simulink model "main_tmp"  (R2021b)
settings: Solver=VariableStepAuto  StartTime=0.0  StopTime=5  FixedStep=Ts  RelTol=1e-3  AbsTol=1e-3  EnableMultiTasking=on
values from neighbouring files (symbols this model uses):
  N = length(dataset.(fldnames{1}))    [create_timeseries.m]    (also in input_data.m = length(t); test_input_data.m = length(t))
undefined symbols (not defined in the file or in its folder): bodyparam, stuffparam, X, Y, Z
libraries: sm_lib x37, nesl_utility x13, Muscles4SimScienceAB x5, Contact_Forces_Lib x2, simulink x1
(part 2 of 2)

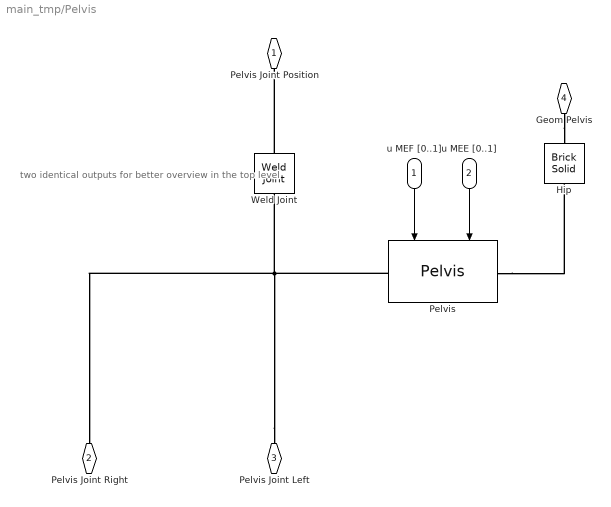
== system main_tmp/Pelvis ==
  note: two identical outputs for better overview in the top level
  u MEF [0..1] : Inport
  u MEE [0..1] : Inport  Port=2
  Hip : sm_lib/Body Elements/Brick Solid  GraphicAmbientColor=[0.15 0.15 0.15 1.0]  BasedOnType=Mass  BrickDimensions=bodyparam.size.hip  BrickDimensionUnits=m  CenterOfMass=[0 0 0]  CenterOfMassUnits=m  GraphicDiffuseColor=[0.5 0.5 0.5]  Density=1000  DensityUnits=kg/m^3  DoExposeReferenceFrame=on  GraphicEmissiveColor=[0.0 0.0 0.0 1.0]  ExportEntireGeometry=on  SerializedFrames=<Frames/>  MarkerShape=Sphere  MarkerSize=10  GraphicType=FromGeometry  InertiaType=Custom  Mass=bodyparam.weight.hip  MassUnits=kg  MomentsOfInertia=[1 1 1]  MomentsOfInertiaUnits=kg*m^2  GraphicOpacity=1.0  ProductsOfInertia=[0 0 0]  ProductsOfInertiaUnits=kg*m^2  GraphicShininess=75  GraphicSpecularColor=[0.5 0.5 0.5 1.0]  GraphicVisPropType=SimpleVisualProperties
  Pelvis : Muscles4SimScienceAB/Pelvis  SystemSampleTime=-1  VariantActivationTime=update diagram  Latency=0  AutoFrameSizeCalculation=off
      settings: SourceProductName=Muscles4SimScienceAB  PortSchema="{\"entries\":[{\"content\":{\"sides\":[{\"content\":{\"connectorIds\":[\"In1\",\"In2\"]},\"type\":\"ConnectorPlacement.EquallySpacedRectSide\",\"uuid\":\"96b1b743-5705-4ec0-abfd-bdeea3d69127\"},{\"content\":{\"connectorIds\":[],\"side\":\"RIGHT\"},\"type\":\"ConnectorPlacement.EquallySpacedRectSide\",\"uuid\":\"b3b1b644-d2fe-42fd-b3a0-cbeacae3e2ea\"},{\"content\":{\"connectorIds\":[\"LConn1\"],\"side\":\"TOP\"},\"type\":\"ConnectorPlacement.EquallySpacedRectSide\",\"uuid\":\"6588cc9c-075c-4f00-8cf7-0671acb35c7c\"},{\"content\":{\"connectorIds\":[\"RConn1\"],\"side\":\"BOTTOM\"},\"type\":\"ConnectorPlacement.EquallySpacedRectSide\",\"uuid\":\"6976fdf2-9376-49cf-8dcb-736f43a1e3aa\"}]},\"type\":\"ConnectorPlacement.EquallySpacedConnector\",\"uuid\":\"9665cf7e-0d90-4f65-9e3e-57dbf89b4304\"}],\"packageUris\":[\"http://schema.mathworks.com/mf0/Connector/R2020b\"],\"version\":\"1.0\"}"
  Weld Joint : sm_lib/Joints/Weld Joint  JointMode=Normal  SenseConstraintForce=off  SenseConstraintForceX=off  SenseConstraintForceY=off  SenseConstraintForceZ=off  SenseConstraintTorque=off  SenseConstraintTorqueX=off  SenseConstraintTorqueY=off  SenseConstraintTorqueZ=off  SenseTotalForce=off  SenseTotalForceX=off  SenseTotalForceY=off  SenseTotalForceZ=off  SenseTotalTorque=off  SenseTotalTorqueX=off  SenseTotalTorqueY=off  SenseTotalTorqueZ=off  CompositeWrenchDir=FollowerOnBase  CompositeWrenchFrame=BaseFrame
  Pelvis Joint Position : PMIOPort  Side=Left
  Pelvis Joint Right : PMIOPort  Port=2  Side=Right
  Pelvis Joint Left : PMIOPort  Port=3  Side=Right
  Geom Pelvis : PMIOPort  Port=4  Side=Right
  wires:
  u MEE [0..1]/1 -> Pelvis/1
  u MEF [0..1]/1 -> Pelvis/2
  connections:
  Weld Joint/RConn1 -- Pelvis Joint Position/RConn1
  Geom Pelvis/RConn1 -- Hip/LConn1
  Pelvis Joint Left/RConn1 -- Pelvis/RConn1 -- Weld Joint/LConn1 -- Pelvis Joint Right/RConn1
  Pelvis/LConn1 -- Hip/RConn1

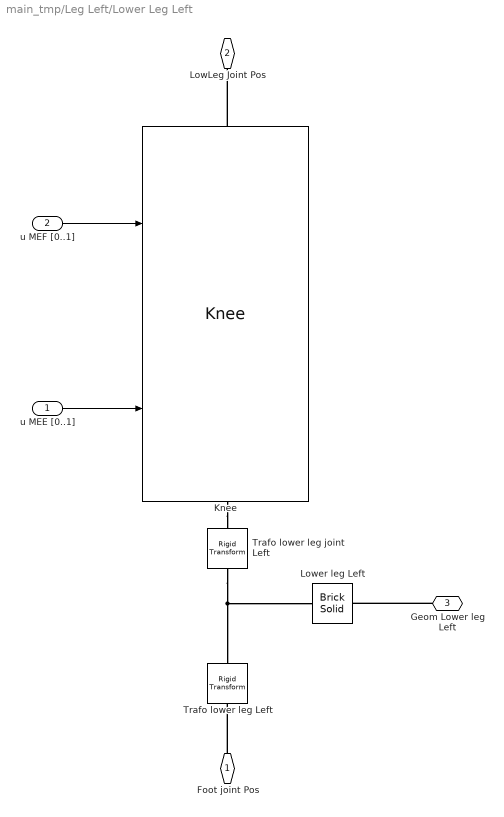
== system main_tmp/Leg Left/Lower Leg Left ==
  u MEE [0..1] : Inport
  u MEF [0..1] : Inport  Port=2
  Knee : Muscles4SimScienceAB/Knee  SystemSampleTime=-1  VariantActivationTime=update diagram  Latency=0  AutoFrameSizeCalculation=off
      settings: SourceProductName=Muscles4SimScienceAB  PortSchema="{\"entries\":[{\"content\":{\"sides\":[{\"content\":{\"connectorIds\":[\"In1\",\"In2\"]},\"type\":\"ConnectorPlacement.EquallySpacedRectSide\",\"uuid\":\"41193043-8a27-4363-8898-1f9e881d08b1\"},{\"content\":{\"connectorIds\":[],\"side\":\"RIGHT\"},\"type\":\"ConnectorPlacement.EquallySpacedRectSide\",\"uuid\":\"5a179196-4a66-423b-80c7-02c9aceed262\"},{\"content\":{\"connectorIds\":[\"LConn1\"],\"side\":\"TOP\"},\"type\":\"ConnectorPlacement.EquallySpacedRectSide\",\"uuid\":\"db447b50-73cc-4af2-8c9c-28a9801561ff\"},{\"content\":{\"connectorIds\":[\"RConn1\"],\"side\":\"BOTTOM\"},\"type\":\"ConnectorPlacement.EquallySpacedRectSide\",\"uuid\":\"bc7ed954-e11d-4420-941c-b14a31097b3c\"}]},\"type\":\"ConnectorPlacement.EquallySpacedConnector\",\"uuid\":\"a73193d2-090f-471b-ad63-2ab894437460\"}],\"packageUris\":[\"http://schema.mathworks.com/mf0/Connector/R2020b\"],\"version\":\"1.0\"}"
  Lower leg Left : sm_lib/Body Elements/Brick Solid  GraphicAmbientColor=[0.15 0.15 0.15 1.0]  BasedOnType=Mass  BrickDimensions=bodyparam.size.lowerleg  BrickDimensionUnits=m  CenterOfMass=[0 0 0]  CenterOfMassUnits=m  GraphicDiffuseColor=[0.2 0.2 1.0]  Density=1000  DensityUnits=kg/m^3  DoExposeReferenceFrame=on  GraphicEmissiveColor=[0.0 0.0 0.0 1.0]  ExportEntireGeometry=on  SerializedFrames=<Frames/>  MarkerShape=Sphere  MarkerSize=10  GraphicType=FromGeometry  InertiaType=Custom  Mass=bodyparam.weight.lowerleg  MassUnits=kg  MomentsOfInertia=[1 1 1]  MomentsOfInertiaUnits=kg*m^2  GraphicOpacity=1.0  ProductsOfInertia=[0 0 0]  ProductsOfInertiaUnits=kg*m^2  GraphicShininess=75  GraphicSpecularColor=[0.5 0.5 0.5 1.0]  GraphicVisPropType=SimpleVisualProperties
  Trafo lower leg Left : sm_lib/Frames and Transforms/Rigid Transform  TranslationMethod=Cartesian  TranslationStandardOffset=0  TranslationLengthUnit=m  TranslationStandardAxis=+Z  TranslationCartesianOffset=bodyparam.position.lowerleg_left_trans.item  TranslationROffset=0  TranslationROffsetUnits=m  TranslationZOffset=0  TranslationZOffsetUnits=m  TranslationThetaOffset=0  TranslationThetaOffsetUnits=deg  RotationMethod=None  RotationAngleUnits=deg  RotationStandardAxis=+Z  RotationAngle=0.0  RotationArbitraryAxis=[0 0 1]  FollAlignAxisA=+X  BaseAlignAxisA=+Y  FollAlignAxisB=+Y  BaseAlignAxisB=+Z  RotationSequenceAxes=FollowerAxes  RotationSequence=XYX  RotationSequenceAngles=[0 0 0]  RotationSequenceAnglesUnits=deg  RotationMatrix=[1 0 0; 0 1 0; 0 0 1]
  Trafo lower leg joint Left : sm_lib/Frames and Transforms/Rigid Transform  TranslationMethod=Cartesian  TranslationStandardOffset=0  TranslationLengthUnit=m  TranslationStandardAxis=+Z  TranslationCartesianOffset=bodyparam.position.lowerleg_left_trans.joint  TranslationROffset=0  TranslationROffsetUnits=m  TranslationZOffset=0  TranslationZOffsetUnits=m  TranslationThetaOffset=0  TranslationThetaOffsetUnits=deg  RotationMethod=None  RotationAngleUnits=deg  RotationStandardAxis=+Z  RotationAngle=0.0  RotationArbitraryAxis=[0 0 1]  FollAlignAxisA=+X  BaseAlignAxisA=+Y  FollAlignAxisB=+Y  BaseAlignAxisB=+Z  RotationSequenceAxes=FollowerAxes  RotationSequence=XYX  RotationSequenceAngles=[0 0 0]  RotationSequenceAnglesUnits=deg  RotationMatrix=[1 0 0; 0 1 0; 0 0 1]
  Foot joint Pos : PMIOPort  Side=Left
  LowLeg Joint Pos : PMIOPort  Port=2  Side=Right
  "Geom Lower leg Left " : PMIOPort  Port=3  Side=Right
  wires:
  u MEE [0..1]/1 -> Knee/2
  u MEF [0..1]/1 -> Knee/1
  connections:
  Trafo lower leg joint Left/LConn1 -- Lower leg Left/RConn1 -- Trafo lower leg Left/RConn1
  Foot joint Pos/RConn1 -- Trafo lower leg Left/LConn1
  Knee/RConn1 -- Trafo lower leg joint Left/RConn1
  Knee/LConn1 -- LowLeg Joint Pos/RConn1
  "Geom Lower leg Left "/RConn1 -- Lower leg Left/LConn1

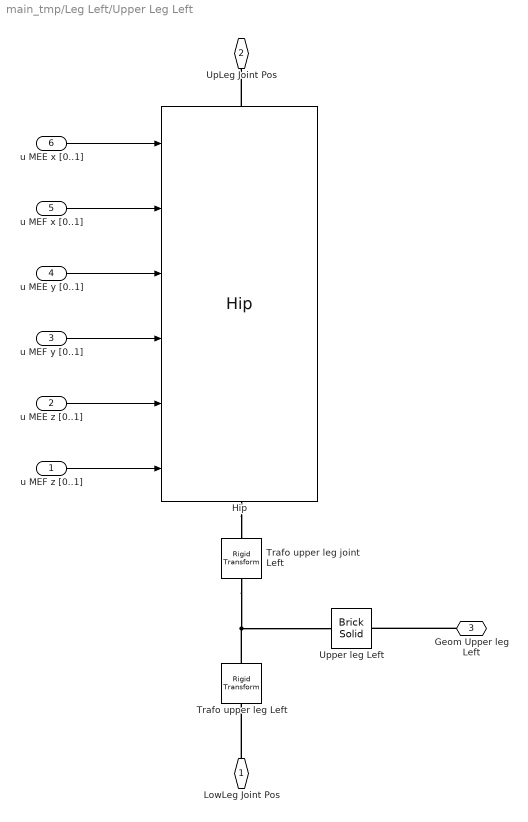
== system main_tmp/Leg Left/Upper Leg Left ==
  u MEF z [0..1] : Inport
  u MEE z [0..1] : Inport  Port=2
  u MEF y [0..1] : Inport  Port=3
  u MEE y [0..1] : Inport  Port=4
  u MEF x [0..1] : Inport  Port=5
  u MEE x [0..1] : Inport  Port=6
  Hip : Muscles4SimScienceAB/Hip  SystemSampleTime=-1  VariantActivationTime=update diagram  Latency=0  AutoFrameSizeCalculation=off
      settings: SourceProductName=Muscles4SimScienceAB  PortSchema="{\"entries\":[{\"content\":{\"sides\":[{\"content\":{\"connectorIds\":[\"In1\",\"In2\",\"In3\",\"In4\",\"In5\",\"In6\"]},\"type\":\"ConnectorPlacement.EquallySpacedRectSide\",\"uuid\":\"41193043-8a27-4363-8898-1f9e881d08b1\"},{\"content\":{\"connectorIds\":[],\"side\":\"RIGHT\"},\"type\":\"ConnectorPlacement.EquallySpacedRectSide\",\"uuid\":\"5a179196-4a66-423b-80c7-02c9aceed262\"},{\"content\":{\"connectorIds\":[\"LConn1\"],\"side\":\"TOP\"},\"type\":\"ConnectorPlacement.EquallySpacedRectSide\",\"uuid\":\"db447b50-73cc-4af2-8c9c-28a9801561ff\"},{\"content\":{\"connectorIds\":[\"RConn1\"],\"side\":\"BOTTOM\"},\"type\":\"ConnectorPlacement.EquallySpacedRectSide\",\"uuid\":\"bc7ed954-e11d-4420-941c-b14a31097b3c\"}]},\"type\":\"ConnectorPlacement.EquallySpacedConnector\",\"uuid\":\"a73193d2-090f-471b-ad63-2ab894437460\"}],\"packageUris\":[\"http://schema.mathworks.com/mf0/Connector/R2020b\"],\"version\":\"1.0\"}"
  Trafo upper leg Left : sm_lib/Frames and Transforms/Rigid Transform  TranslationMethod=Cartesian  TranslationStandardOffset=0  TranslationLengthUnit=m  TranslationStandardAxis=+Z  TranslationCartesianOffset=bodyparam.position.upperleg_left_trans.item  TranslationROffset=0  TranslationROffsetUnits=m  TranslationZOffset=0  TranslationZOffsetUnits=m  TranslationThetaOffset=0  TranslationThetaOffsetUnits=deg  RotationMethod=None  RotationAngleUnits=deg  RotationStandardAxis=+Z  RotationAngle=0.0  RotationArbitraryAxis=[0 0 1]  FollAlignAxisA=+X  BaseAlignAxisA=+Y  FollAlignAxisB=+Y  BaseAlignAxisB=+Z  RotationSequenceAxes=FollowerAxes  RotationSequence=XYX  RotationSequenceAngles=[0 0 0]  RotationSequenceAnglesUnits=deg  RotationMatrix=[1 0 0; 0 1 0; 0 0 1]
  Trafo upper leg joint Left : sm_lib/Frames and Transforms/Rigid Transform  TranslationMethod=Cartesian  TranslationStandardOffset=0  TranslationLengthUnit=m  TranslationStandardAxis=+Z  TranslationCartesianOffset=bodyparam.position.upperleg_left_trans.joint  TranslationROffset=0  TranslationROffsetUnits=m  TranslationZOffset=0  TranslationZOffsetUnits=m  TranslationThetaOffset=0  TranslationThetaOffsetUnits=deg  RotationMethod=None  RotationAngleUnits=deg  RotationStandardAxis=+Z  RotationAngle=0.0  RotationArbitraryAxis=[0 0 1]  FollAlignAxisA=+X  BaseAlignAxisA=+Y  FollAlignAxisB=+Y  BaseAlignAxisB=+Z  RotationSequenceAxes=FollowerAxes  RotationSequence=XYX  RotationSequenceAngles=[0 0 0]  RotationSequenceAnglesUnits=deg  RotationMatrix=[1 0 0; 0 1 0; 0 0 1]
  Upper leg Left : sm_lib/Body Elements/Brick Solid  GraphicAmbientColor=[0.15 0.15 0.15 1.0]  BasedOnType=Mass  BrickDimensions=bodyparam.size.upperleg  BrickDimensionUnits=m  CenterOfMass=[0 0 0]  CenterOfMassUnits=m  GraphicDiffuseColor=[0.5 0.5 0.5]  Density=1000  DensityUnits=kg/m^3  DoExposeReferenceFrame=on  GraphicEmissiveColor=[0.0 0.0 0.0 1.0]  ExportEntireGeometry=on  SerializedFrames=<Frames/>  MarkerShape=Sphere  MarkerSize=10  GraphicType=FromGeometry  InertiaType=Custom  Mass=bodyparam.weight.upperleg  MassUnits=kg  MomentsOfInertia=[1 1 1]  MomentsOfInertiaUnits=kg*m^2  GraphicOpacity=1.0  ProductsOfInertia=[0 0 0]  ProductsOfInertiaUnits=kg*m^2  GraphicShininess=75  GraphicSpecularColor=[0.5 0.5 0.5 1.0]  GraphicVisPropType=SimpleVisualProperties
  LowLeg Joint Pos : PMIOPort  Side=Left
  UpLeg Joint Pos : PMIOPort  Port=2  Side=Right
  "Geom Upper leg Left " : PMIOPort  Port=3  Side=Right
  wires:
  u MEE z [0..1]/1 -> Hip/5
  u MEE x [0..1]/1 -> Hip/1
  u MEF x [0..1]/1 -> Hip/2
  u MEF z [0..1]/1 -> Hip/6
  u MEE y [0..1]/1 -> Hip/3
  u MEF y [0..1]/1 -> Hip/4
  connections:
  Hip/LConn1 -- UpLeg Joint Pos/RConn1
  LowLeg Joint Pos/RConn1 -- Trafo upper leg Left/LConn1
  Trafo upper leg Left/RConn1 -- Trafo upper leg joint Left/LConn1 -- Upper leg Left/RConn1
  Hip/RConn1 -- Trafo upper leg joint Left/RConn1
  "Geom Upper leg Left "/RConn1 -- Upper leg Left/LConn1

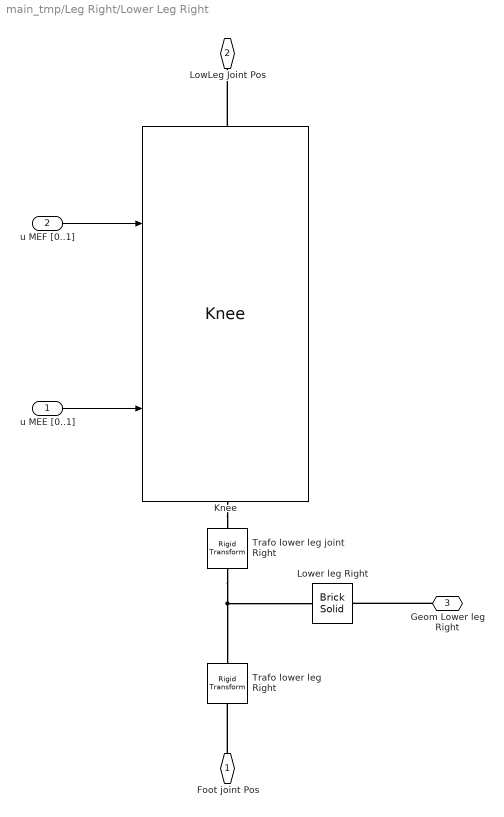
== system main_tmp/Leg Right/Lower Leg Right ==
  u MEE [0..1] : Inport
  u MEF [0..1] : Inport  Port=2
  Knee : Muscles4SimScienceAB/Knee  SystemSampleTime=-1  VariantActivationTime=update diagram  Latency=0  AutoFrameSizeCalculation=off
      settings: SourceProductName=Muscles4SimScienceAB  PortSchema="{\"entries\":[{\"content\":{\"sides\":[{\"content\":{\"connectorIds\":[\"In1\",\"In2\"]},\"type\":\"ConnectorPlacement.EquallySpacedRectSide\",\"uuid\":\"41193043-8a27-4363-8898-1f9e881d08b1\"},{\"content\":{\"connectorIds\":[],\"side\":\"RIGHT\"},\"type\":\"ConnectorPlacement.EquallySpacedRectSide\",\"uuid\":\"5a179196-4a66-423b-80c7-02c9aceed262\"},{\"content\":{\"connectorIds\":[\"LConn1\"],\"side\":\"TOP\"},\"type\":\"ConnectorPlacement.EquallySpacedRectSide\",\"uuid\":\"db447b50-73cc-4af2-8c9c-28a9801561ff\"},{\"content\":{\"connectorIds\":[\"RConn1\"],\"side\":\"BOTTOM\"},\"type\":\"ConnectorPlacement.EquallySpacedRectSide\",\"uuid\":\"bc7ed954-e11d-4420-941c-b14a31097b3c\"}]},\"type\":\"ConnectorPlacement.EquallySpacedConnector\",\"uuid\":\"a73193d2-090f-471b-ad63-2ab894437460\"}],\"packageUris\":[\"http://schema.mathworks.com/mf0/Connector/R2020b\"],\"version\":\"1.0\"}"
  Lower leg Right : sm_lib/Body Elements/Brick Solid  GraphicAmbientColor=[0.15 0.15 0.15 1.0]  BasedOnType=Mass  BrickDimensions=bodyparam.size.lowerleg  BrickDimensionUnits=m  CenterOfMass=[0 0 0]  CenterOfMassUnits=m  GraphicDiffuseColor=[0.2 0.2 1.0]  Density=1000  DensityUnits=kg/m^3  DoExposeReferenceFrame=on  GraphicEmissiveColor=[0.0 0.0 0.0 1.0]  ExportEntireGeometry=on  SerializedFrames=<Frames/>  MarkerShape=Sphere  MarkerSize=10  GraphicType=FromGeometry  InertiaType=Custom  Mass=bodyparam.weight.lowerleg  MassUnits=kg  MomentsOfInertia=[1 1 1]  MomentsOfInertiaUnits=kg*m^2  GraphicOpacity=1.0  ProductsOfInertia=[0 0 0]  ProductsOfInertiaUnits=kg*m^2  GraphicShininess=75  GraphicSpecularColor=[0.5 0.5 0.5 1.0]  GraphicVisPropType=SimpleVisualProperties
  Trafo lower leg Right : sm_lib/Frames and Transforms/Rigid Transform  TranslationMethod=Cartesian  TranslationStandardOffset=0  TranslationLengthUnit=m  TranslationStandardAxis=+Z  TranslationCartesianOffset=bodyparam.position.lowerleg_right_trans.item  TranslationROffset=0  TranslationROffsetUnits=m  TranslationZOffset=0  TranslationZOffsetUnits=m  TranslationThetaOffset=0  TranslationThetaOffsetUnits=deg  RotationMethod=None  RotationAngleUnits=deg  RotationStandardAxis=+Z  RotationAngle=0.0  RotationArbitraryAxis=[0 0 1]  FollAlignAxisA=+X  BaseAlignAxisA=+Y  FollAlignAxisB=+Y  BaseAlignAxisB=+Z  RotationSequenceAxes=FollowerAxes  RotationSequence=XYX  RotationSequenceAngles=[0 0 0]  RotationSequenceAnglesUnits=deg  RotationMatrix=[1 0 0; 0 1 0; 0 0 1]
  Trafo lower leg joint Right : sm_lib/Frames and Transforms/Rigid Transform  TranslationMethod=Cartesian  TranslationStandardOffset=0  TranslationLengthUnit=m  TranslationStandardAxis=+Z  TranslationCartesianOffset=bodyparam.position.lowerleg_right_trans.joint  TranslationROffset=0  TranslationROffsetUnits=m  TranslationZOffset=0  TranslationZOffsetUnits=m  TranslationThetaOffset=0  TranslationThetaOffsetUnits=deg  RotationMethod=None  RotationAngleUnits=deg  RotationStandardAxis=+Z  RotationAngle=0.0  RotationArbitraryAxis=[0 0 1]  FollAlignAxisA=+X  BaseAlignAxisA=+Y  FollAlignAxisB=+Y  BaseAlignAxisB=+Z  RotationSequenceAxes=FollowerAxes  RotationSequence=XYX  RotationSequenceAngles=[0 0 0]  RotationSequenceAnglesUnits=deg  RotationMatrix=[1 0 0; 0 1 0; 0 0 1]
  Foot joint Pos : PMIOPort  Side=Left
  LowLeg Joint Pos : PMIOPort  Port=2  Side=Right
  "Geom Lower leg Right " : PMIOPort  Port=3  Side=Right
  wires:
  u MEE [0..1]/1 -> Knee/2
  u MEF [0..1]/1 -> Knee/1
  connections:
  Trafo lower leg joint Right/LConn1 -- Lower leg Right/RConn1 -- Trafo lower leg Right/RConn1
  Foot joint Pos/RConn1 -- Trafo lower leg Right/LConn1
  Knee/RConn1 -- Trafo lower leg joint Right/RConn1
  Knee/LConn1 -- LowLeg Joint Pos/RConn1
  "Geom Lower leg Right "/RConn1 -- Lower leg Right/LConn1

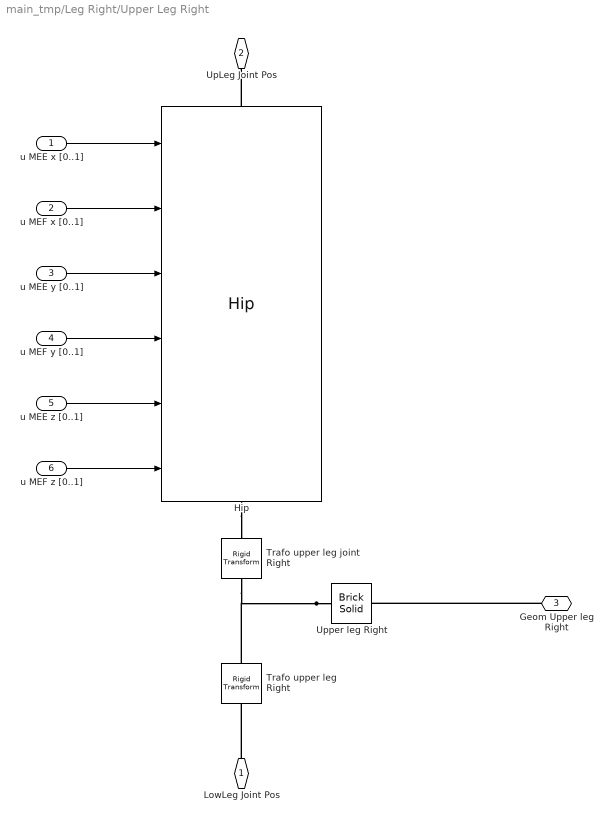
== system main_tmp/Leg Right/Upper Leg Right ==
  u MEE x [0..1] : Inport
  u MEF x [0..1] : Inport  Port=2
  u MEE y [0..1] : Inport  Port=3
  u MEF y [0..1] : Inport  Port=4
  u MEE z [0..1] : Inport  Port=5
  u MEF z [0..1] : Inport  Port=6
  Hip : Muscles4SimScienceAB/Hip  SystemSampleTime=-1  VariantActivationTime=update diagram  Latency=0  AutoFrameSizeCalculation=off
      settings: SourceProductName=Muscles4SimScienceAB  PortSchema="{\"entries\":[{\"content\":{\"sides\":[{\"content\":{\"connectorIds\":[\"In1\",\"In2\",\"In3\",\"In4\",\"In5\",\"In6\"]},\"type\":\"ConnectorPlacement.EquallySpacedRectSide\",\"uuid\":\"41193043-8a27-4363-8898-1f9e881d08b1\"},{\"content\":{\"connectorIds\":[],\"side\":\"RIGHT\"},\"type\":\"ConnectorPlacement.EquallySpacedRectSide\",\"uuid\":\"5a179196-4a66-423b-80c7-02c9aceed262\"},{\"content\":{\"connectorIds\":[\"LConn1\"],\"side\":\"TOP\"},\"type\":\"ConnectorPlacement.EquallySpacedRectSide\",\"uuid\":\"db447b50-73cc-4af2-8c9c-28a9801561ff\"},{\"content\":{\"connectorIds\":[\"RConn1\"],\"side\":\"BOTTOM\"},\"type\":\"ConnectorPlacement.EquallySpacedRectSide\",\"uuid\":\"bc7ed954-e11d-4420-941c-b14a31097b3c\"}]},\"type\":\"ConnectorPlacement.EquallySpacedConnector\",\"uuid\":\"a73193d2-090f-471b-ad63-2ab894437460\"}],\"packageUris\":[\"http://schema.mathworks.com/mf0/Connector/R2020b\"],\"version\":\"1.0\"}"
  Trafo upper leg Right : sm_lib/Frames and Transforms/Rigid Transform  TranslationMethod=Cartesian  TranslationStandardOffset=0  TranslationLengthUnit=m  TranslationStandardAxis=+Z  TranslationCartesianOffset=bodyparam.position.upperleg_right_trans.item  TranslationROffset=0  TranslationROffsetUnits=m  TranslationZOffset=0  TranslationZOffsetUnits=m  TranslationThetaOffset=0  TranslationThetaOffsetUnits=deg  RotationMethod=None  RotationAngleUnits=deg  RotationStandardAxis=+Z  RotationAngle=0.0  RotationArbitraryAxis=[0 0 1]  FollAlignAxisA=+X  BaseAlignAxisA=+Y  FollAlignAxisB=+Y  BaseAlignAxisB=+Z  RotationSequenceAxes=FollowerAxes  RotationSequence=XYX  RotationSequenceAngles=[0 0 0]  RotationSequenceAnglesUnits=deg  RotationMatrix=[1 0 0; 0 1 0; 0 0 1]
  Trafo upper leg joint Right : sm_lib/Frames and Transforms/Rigid Transform  TranslationMethod=Cartesian  TranslationStandardOffset=0  TranslationLengthUnit=m  TranslationStandardAxis=+Z  TranslationCartesianOffset=bodyparam.position.upperleg_right_trans.joint  TranslationROffset=0  TranslationROffsetUnits=m  TranslationZOffset=0  TranslationZOffsetUnits=m  TranslationThetaOffset=0  TranslationThetaOffsetUnits=deg  RotationMethod=None  RotationAngleUnits=deg  RotationStandardAxis=+Z  RotationAngle=0.0  RotationArbitraryAxis=[0 0 1]  FollAlignAxisA=+X  BaseAlignAxisA=+Y  FollAlignAxisB=+Y  BaseAlignAxisB=+Z  RotationSequenceAxes=FollowerAxes  RotationSequence=XYX  RotationSequenceAngles=[0 0 0]  RotationSequenceAnglesUnits=deg  RotationMatrix=[1 0 0; 0 1 0; 0 0 1]
  Upper leg Right : sm_lib/Body Elements/Brick Solid  GraphicAmbientColor=[0.15 0.15 0.15 1.0]  BasedOnType=Mass  BrickDimensions=bodyparam.size.upperleg  BrickDimensionUnits=m  CenterOfMass=[0 0 0]  CenterOfMassUnits=m  GraphicDiffuseColor=[0.5 0.5 0.5]  Density=1000  DensityUnits=kg/m^3  DoExposeReferenceFrame=on  GraphicEmissiveColor=[0.0 0.0 0.0 1.0]  ExportEntireGeometry=on  SerializedFrames=<Frames/>  MarkerShape=Sphere  MarkerSize=10  GraphicType=FromGeometry  InertiaType=Custom  Mass=bodyparam.weight.upperleg  MassUnits=kg  MomentsOfInertia=[1 1 1]  MomentsOfInertiaUnits=kg*m^2  GraphicOpacity=1.0  ProductsOfInertia=[0 0 0]  ProductsOfInertiaUnits=kg*m^2  GraphicShininess=75  GraphicSpecularColor=[0.5 0.5 0.5 1.0]  GraphicVisPropType=SimpleVisualProperties
  LowLeg Joint Pos : PMIOPort  Side=Left
  UpLeg Joint Pos : PMIOPort  Port=2  Side=Right
  "Geom Upper leg Right " : PMIOPort  Port=3  Side=Right
  wires:
  u MEE y [0..1]/1 -> Hip/3
  u MEF z [0..1]/1 -> Hip/6
  u MEE z [0..1]/1 -> Hip/5
  u MEF y [0..1]/1 -> Hip/4
  u MEF x [0..1]/1 -> Hip/2
  u MEE x [0..1]/1 -> Hip/1
  connections:
  Upper leg Right/RConn1 -- Trafo upper leg Right/RConn1 -- Trafo upper leg joint Right/LConn1
  LowLeg Joint Pos/RConn1 -- Trafo upper leg Right/LConn1
  Hip/LConn1 -- UpLeg Joint Pos/RConn1
  Hip/RConn1 -- Trafo upper leg joint Right/RConn1
  "Geom Upper leg Right "/RConn1 -- Upper leg Right/LConn1
